simulink model "W_server_oClientServer_Model"  (R2024b)
settings: Solver=FixedStepDiscrete  StartTime=0.0  StopTime=10.0  FixedStep=0.05  RelTol=1e-3
settings Model: Tag=EP_AA_WRAPPER_SERVER  DataDictionary=Wrapper_oClientServer_Model.sldd  Creator=nabilekhoury  LastModifiedBy=nabilekhoury
settings OptimizationCC: DefaultParameterBehavior=Inlined  OptimizeBlockIOStorage=off  BufferReuse=off  ReuseModelBlockBuffer=off  GlobalBufferReuse=off  ExpressionFolding=off  EnableMemcpy=off  PassReuseOutputArgsAs=Individual arguments  LocalBlockOutputs=off  ZeroExternalMemoryAtStartup=off  ZeroInternalMemoryAtStartup=off  OptimizeDataStoreBuffers=off  BusAssignmentInplaceUpdate=off  OptimizationLevel=level0  OptimizationCustomize=off  EfficientTunableParamExpr=on
settings DebuggingCC: ParameterTunabilityLossMsg=error
settings ModelReferenceCC: ModelReferenceNumInstancesAllowed=Single
settings SFSimCC: MATLABDynamicMemAlloc=off  SimTargetLang=C++
settings RTWCC: Description=Embedded Coder  SystemTargetFile=ert.tlc  GenCodeOnly=on  TemplateMakefile=ert_default_tmf  CustomSourceCode="#include \"oClientServer_Model_adapter.h\""  CustomInitializer=sut_initialize();  TargetLang=C++
settings CodeAppCC: ForceParamTrailComments=on  IgnoreCustomStorageClasses=off  MaxIdLength=256  OperatorAnnotations=on  SimulinkDataObjDesc=on  SFDataObjDesc=on  CustomSymbolStrGlobalVar=w_$R$N$M  CustomSymbolStrType=w_$N$R$M_T  InsertBlockDesc=on
settings ERTTargetCC: TargetLangStandard=C++17 (ISO)  GenerateSampleERTMain=on  SupportAbsoluteTime=off  SupportNonFinite=off  SupportComplex=off  RootIOFormat=Structure reference  ERTCustomFileTemplate=example_file_process.tlc

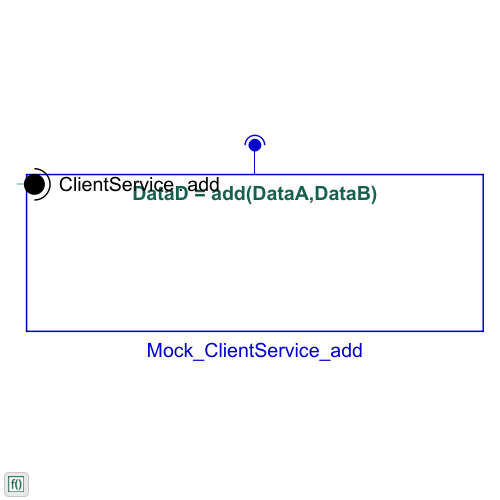
[thumbnail: Simulink's stored preview of the top-level diagram]
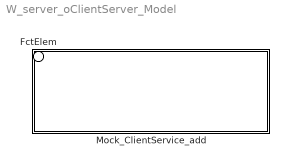
== system W_server_oClientServer_Model ==
  Mock_ClientService_add : Subsystem  TreatAsAtomicUnit=on
  FctElem : Outport  AllowServiceAccess=on  PortName=ClientService  Element=add

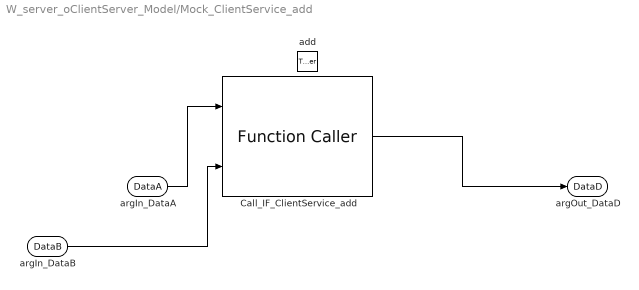
== system W_server_oClientServer_Model/Mock_ClientService_add ==
  add : TriggerPort  TriggerType=function-call  IsSimulinkFunction=on  FunctionName=add  FunctionVisibility=port  ScopeName=ClientService  VariantControl=(inherit)
  Call_IF_ClientService_add : FunctionCaller  FunctionPrototype=DataD = IF_ClientService_add(DataA,DataB)  InputArgumentSpecifications=double(0), double(0)  OutputArgumentSpecifications=double(0)
  argIn_DataA : ArgIn  PortDimensions=[1 1]  ArgumentName=DataA
  argIn_DataB : ArgIn  Port=2  PortDimensions=[1 1]  ArgumentName=DataB
  argOut_DataD : ArgOut  PortDimensions=[1 1]  ArgumentName=DataD
  wires:
  argIn_DataA/1 -> Call_IF_ClientService_add/1
  argIn_DataB/1 -> Call_IF_ClientService_add/2
  Call_IF_ClientService_add/1 -> argOut_DataD/1
